simulink model "PMSM_standAlone_Dev"  (R2023b)
settings: Solver=ode4  StartTime=0.0  StopTime=2  FixedStep=1e-4  RelTol=1e-3
values from neighbouring files (symbols this model uses):
  Ki = BW*rs    (= 12.5663706144)    [PI_parameters_STEADY_STATE_ROTOR_REFERANCED_PMSM.m]
  Kp = BW*Lq    (= 0.0188495559215)    [PI_parameters_STEADY_STATE_ROTOR_REFERANCED_PMSM.m]
settings Model: Creator=szymo  LastModifiedBy=szymo

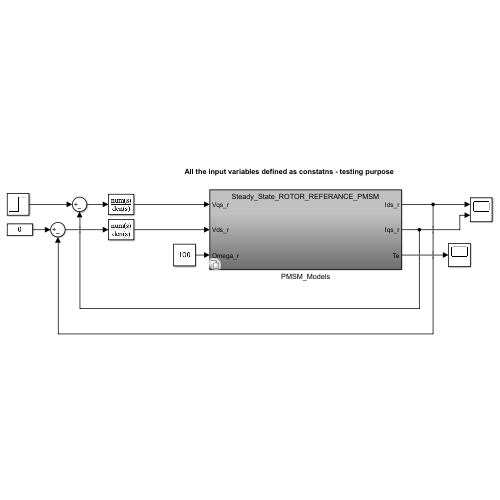
[thumbnail: Simulink's stored preview of the top-level diagram]
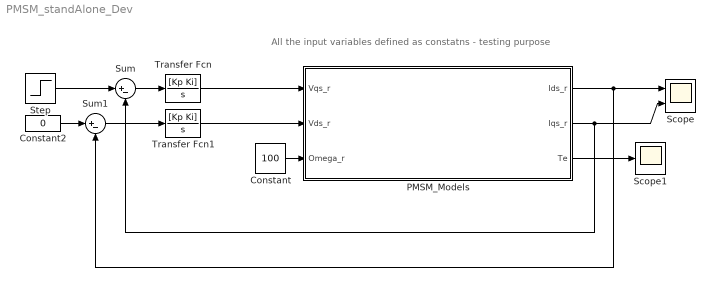
== system PMSM_standAlone_Dev ==
  note: All the input variables defined as constatns - testing purpose
  Constant : Constant  Value=100
  Constant2 : Constant  Value=0
  PMSM_Models : Subsystem  Variant=on
  Scope : Scope  NumInputPorts=2
  Scope1 : Scope
  Step : Step  After=2  SampleTime=0
  Sum : Sum  Inputs=|+-
  Sum1 : Sum  Inputs=|+-
  Transfer Fcn : TransferFcn  Numerator=[Kp Ki]  Denominator=[1 0]
  Transfer Fcn1 : TransferFcn  Numerator=[Kp Ki]  Denominator=[1 0]
  wires:
  Constant/1 -> PMSM_Models/3(Omega_r)
  PMSM_Models/1(Ids_r) -> Sum1/2, Scope/1
  PMSM_Models/2(Iqs_r) -> Sum/2, Scope/2
  PMSM_Models/3(Te) -> Scope1/1
  Transfer Fcn/1 -> PMSM_Models/1(Vqs_r)
  Transfer Fcn1/1 -> PMSM_Models/2(Vds_r)
  Constant2/1 -> Sum1/1
  Sum1/1 -> Transfer Fcn1/1
  Step/1 -> Sum/1
  Sum/1 -> Transfer Fcn/1

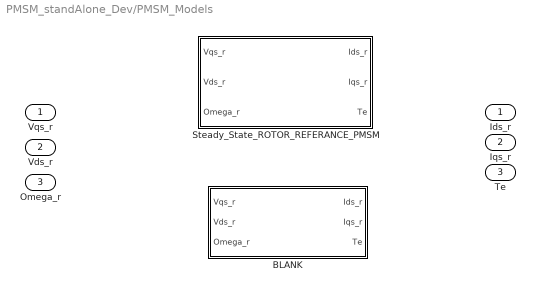
== system PMSM_standAlone_Dev/PMSM_Models ==
  Vqs_r : Inport
  Vds_r : Inport  Port=2
  Omega_r : Inport  Port=3
  BLANK : Subsystem  VariantControl=Model==2
  Steady_State_ROTOR_REFERANCE_PMSM : Subsystem  VariantControl=Model==1
  Ids_r : Outport
  Iqs_r : Outport  Port=2
  Te : Outport  Port=3

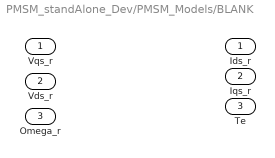
== system PMSM_standAlone_Dev/PMSM_Models/BLANK ==
  Vqs_r : Inport
  Vds_r : Inport  Port=2
  Omega_r : Inport  Port=3
  Ids_r : Outport
  Iqs_r : Outport  Port=2
  Te : Outport  Port=3

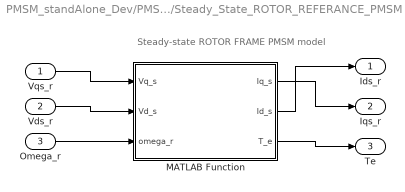
== system PMSM_standAlone_Dev/PMSM_Models/Steady_State_ROTOR_REFERANCE_PMSM ==
  note: Steady-state ROTOR FRAME PMSM model
  Vqs_r : Inport
  Vds_r : Inport  Port=2
  Omega_r : Inport  Port=3
  MATLAB Function : MATLAB Function  TreatAsAtomicUnit=on
  Ids_r : Outport
  Iqs_r : Outport  Port=2
  Te : Outport  Port=3
  wires:
  Vqs_r/1 -> MATLAB Function/1(Vq_s)
  Vds_r/1 -> MATLAB Function/2(Vd_s)
  Omega_r/1 -> MATLAB Function/3(omega_r)
  MATLAB Function/3(T_e) -> Te/1
  MATLAB Function/1(Iq_s) -> Iqs_r/1
  MATLAB Function/2(Id_s) -> Ids_r/1

== matlab function PMSM_standAlone_Dev/PMSM_Models/Steady_State_ROTOR_REFERANCE_PMSM/MATLAB Function ==
  data: Vq_s input; Iq_s output; Id_s output; T_e output; Vd_s input; omega_r input
function [Iq_s, Id_s, T_e] = fcn(Vq_s, Vd_s, omega_r)

%Physical constans of the PMSM - steady state
rs = 0.2;
Lq = 300e-6;
Ld = 300e-6;
Lambda_m_r = 0.01;
P = 2; %Poles (one pole pair)


%Evaluation of DC currents for d and q axis and torque 
K1 = ((rs^2)+(omega_r^2)*Lq*Ld);

Iq_s = (rs/K1)*(Vq_s-omega_r*Lambda_m_r-(omega_r*Ld/rs)*Vd_s);
Id_s = (1/K1)*(rs*Vd_s+omega_r*Lq*Vq_s-(omega_r^2)*Lq*Lambda_m_r);

T_e = (3/2)*(P/2)*(Lambda_m_r*Iq_s+(Ld-Lq)*Iq_s*Id_s);

end
